simulink model "Control_system"  (R2020a)
settings: Solver=ode45  StartTime=0.0  StopTime=tfinal  RelTol=1e-6  EnableMultiTasking=on
values from neighbouring files (symbols this model uses):
  A = [5.13674577679 1 0 0 0 0 -11.4974040302 0 1 0 0 0 ... (36 elements, 6x6)]    [state_space_model.mat]
  B = [1 0 0 0 0 0]    [state_space_model.mat]
  C = [0 -8.56427886647e-05 0.000639852636745 -0.000603207268883 0 0]    [state_space_model.mat]
  Nbar = Nu+K*Nx    [Control_script.m]
  Ts = 1/fs    (= 0.01)    [Control_script.m]
undefined symbols (not defined in the file or in its folder): Atrue, Btrue, Ctrue, Dtrue, K
settings Model: Creator=jomle  LastModifiedBy=franc
settings DataIOCC: LimitDataPoints=on  SaveFormat=Array  ReturnWorkspaceOutputs=off
settings OptimizationCC: LifeSpan=inf
settings DebuggingCC: SFUnexpectedBacktrackingDiag=warning  SFNoUnconditionalDefaultTransitionDiag=warning  SFExecutionAtInitializationDiag=none  ArithmeticOperatorsInVariantConditions=warning
settings HardwareCC: ProdBitPerPointer=32  ProdBitPerSizeT=32  ProdBitPerPtrDiffT=32  ProdLargestAtomicFloat=None  ProdIntDivRoundTo=Undefined  ProdEndianess=Unspecified  ProdWordSize=32  ProdHWDeviceType=32-bit Generic
settings ModelReferenceCC: PropagateSignalLabelsOutOfModel=off
settings SFSimCC: SimUseLocalCustomCode=off  CustomCodeUndefinedFunction=UseInterfaceOnly
settings RTWCC: RTWUseLocalCustomCode=off
settings CodeAppCC: StateflowObjectComments=on
settings GRTTargetCC: TargetLangStandard=C89/C90 (ANSI)
settings ConfigComp: CovMetricSettings=dw  CovHtmlReporting=on  CovSaveCumulativeToWorkspaceVar=on  CovSaveSingleToWorkspaceVar=on  CovExternalEMLEnable=off

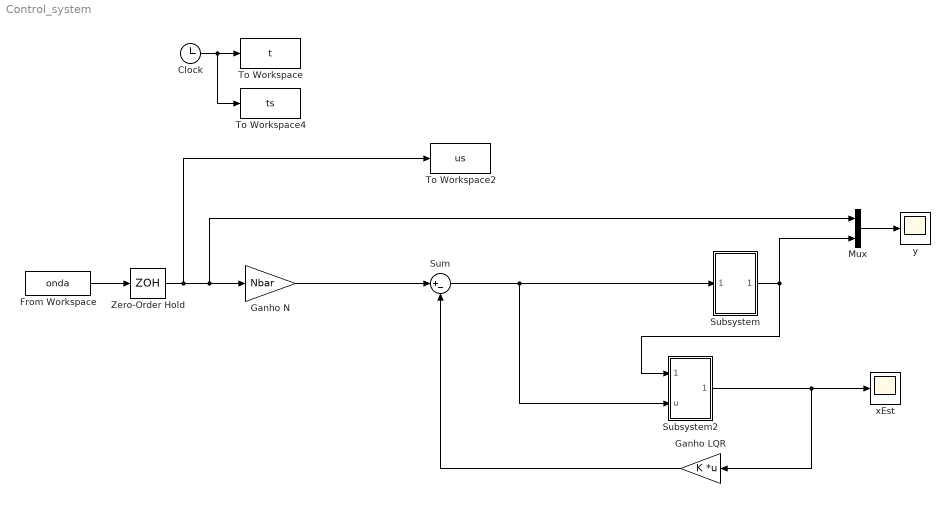
== system Control_system ==
  Clock : Clock
  From Workspace : FromWorkspace  VariableName=onda
  Ganho LQR : Gain  Gain=K  Multiplication=Matrix(K*u)
  Ganho N : Gain  Gain=Nbar
  Mux : Mux  Inputs=2
  Subsystem : Subsystem
  Subsystem2 : Subsystem
  Sum : Sum  Inputs=|+-
  To Workspace : ToWorkspace  VariableName=t  SampleTime=-1
  To Workspace2 : ToWorkspace  VariableName=us  SampleTime=Ts
  To Workspace4 : ToWorkspace  VariableName=ts  SampleTime=Ts
  Zero-Order Hold : ZeroOrderHold  SampleTime=Ts
  xEst : Scope
  y : Scope
  wires:
  Clock/1 -> To Workspace4/1, To Workspace/1
  Zero-Order Hold/1 -> Ganho N/1, Mux/1, To Workspace2/1
  From Workspace/1 -> Zero-Order Hold/1
  Sum/1 -> Subsystem2/2(u), Subsystem/1(In1)
  Ganho LQR/1 -> Sum/2
  Mux/1 -> y/1
  Subsystem/1(y_mod) -> Subsystem2/1(y_mod), Mux/2
  Ganho N/1 -> Sum/1
  Subsystem2/1(x_est) -> Ganho LQR/1, xEst/1

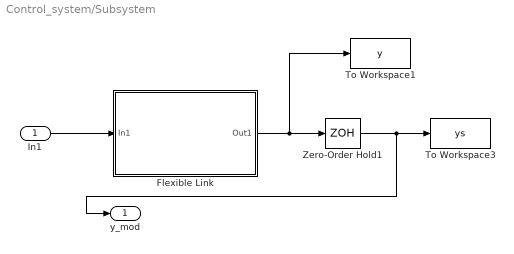
== system Control_system/Subsystem ==
  In1 : Inport
  Flexible Link : Subsystem
      mask Display: image('quanserlink.jpg')
  To Workspace1 : ToWorkspace  VariableName=y  SampleTime=-1
  To Workspace3 : ToWorkspace  VariableName=ys  SampleTime=Ts
  Zero-Order Hold1 : ZeroOrderHold  SampleTime=Ts
  y_mod : Outport
  wires:
  Flexible Link/1(Out1) -> Zero-Order Hold1/1, To Workspace1/1
  In1/1 -> Flexible Link/1(In1)
  Zero-Order Hold1/1 -> y_mod/1, To Workspace3/1

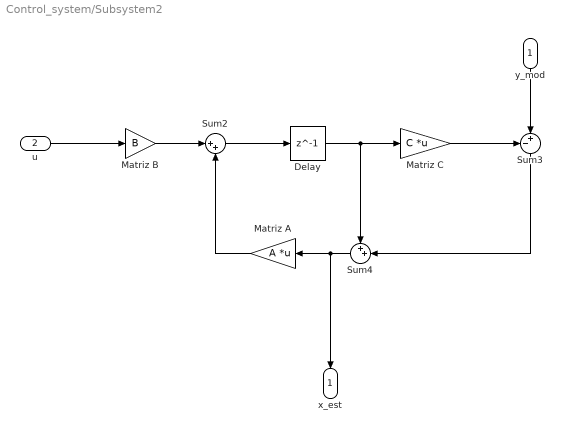
== system Control_system/Subsystem2 ==
  y_mod : Inport
  u : Inport  Port=2
  Delay : Delay  DelayLength=1  InitialCondition=0
  Matriz A : Gain  Gain=A  Multiplication=Matrix(K*u)
  Matriz B : Gain  Gain=B
  Matriz C : Gain  Gain=C  Multiplication=Matrix(K*u)
  Sum2 : Sum  Inputs=|++
  Sum3 : Sum  Inputs=-+|
  Sum4 : Sum  Inputs=++|
  x_est : Outport  VectorParamsAs1DForOutWhenUnconnected=off
  wires:
  Sum3/1 -> Sum4/2
  Sum4/1 -> x_est/1, Matriz A/1
  Sum2/1 -> Delay/1
  y_mod/1 -> Sum3/2
  Matriz B/1 -> Sum2/1
  Matriz A/1 -> Sum2/2
  u/1 -> Matriz B/1
  Matriz C/1 -> Sum3/1
  Delay/1 -> Sum4/1, Matriz C/1

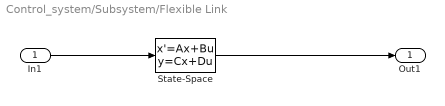
== system Control_system/Subsystem/Flexible Link ==
  In1 : Inport
  State-Space : StateSpace  A=Atrue  B=Btrue  C=Ctrue  D=Dtrue  InitialCondition=0
  Out1 : Outport
  wires:
  State-Space/1 -> Out1/1
  In1/1 -> State-Space/1
